simulink model "pi_linear_model"  (R2015a)
settings: Solver=ode45  StartTime=0.0  StopTime=10  RelTol=1e-3
settings Model: Creator=Home  LastModifiedBy=Home

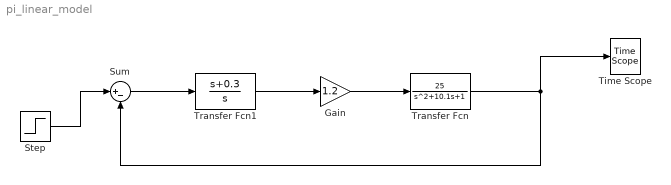
== system pi_linear_model ==
  Gain : Gain  Gain=1.2
  Step : Step  Time=0  After=50  SampleTime=0
  Sum : Sum  Inputs=|+-
  Time Scope : TimeScope  DefaultConfigurationName=spbscopes.TimeScopeBlockCfg
  Transfer Fcn : TransferFcn  Numerator=[25]  Denominator=[1 10.1 1]
  Transfer Fcn1 : TransferFcn  Numerator=[1 0.3]  Denominator=[1 0]
  wires:
  Step/1 -> Sum/1
  Sum/1 -> Transfer Fcn1/1
  Transfer Fcn1/1 -> Gain/1
  Gain/1 -> Transfer Fcn/1
  Transfer Fcn/1 -> Sum/2, Time Scope/1
